simulink model "PID_Controller_referencedModel"  (R2021b)
settings: Solver=VariableStepAuto  StartTime=0.0  StopTime=10.0  RelTol=1e-3
model mask{Ki=Ki, Kp=Kp}
model workspace (MAT data in the model file):
  Kd = 1
  Ki = 1
  Kp = 1000
  Ts = 0.01
settings Model: ParameterArgumentNames=Ki,Kp  Creator=vigne  LastModifiedBy=vigne
settings DataIOCC: SaveOutput=off  SaveTime=off

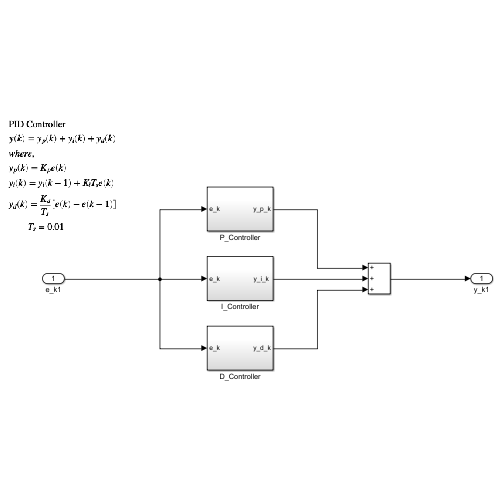
[thumbnail: Simulink's stored preview of the top-level diagram]
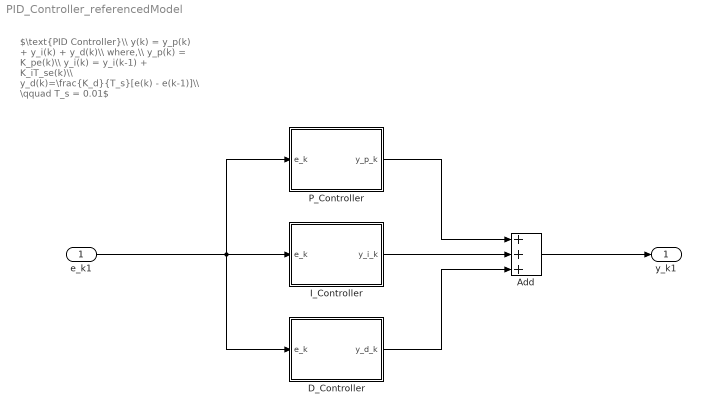
== system PID_Controller_referencedModel ==
  note: $\text{PID Controller}\\ y(k) = y_p(k) + y_i(k) + y_d(k)\\ where,\\ y_p(k) = K_pe(k)\\ y_i(k) = y_i(k-1) + K_iT_se(k)\\ y_d(k)=\frac{K_d}{T_s}[e(k) - e(k-1)]\\ \qquad T_s = 0.01$
  e_k1 : Inport  OutDataTypeStr=double  PortDimensions=1  SampleTime=0
  Add : Sum  Inputs=+++
  D_Controller : Subsystem
  I_Controller : Subsystem
  P_Controller : Subsystem
  y_k1 : Outport  OutDataTypeStr=double  PortDimensions=1  SampleTime=0
  wires:
  D_Controller/1(y_d_k) -> Add/3
  P_Controller/1(y_p_k) -> Add/1
  e_k1/1 -> P_Controller/1(e_k), D_Controller/1(e_k), I_Controller/1(e_k)
  I_Controller/1("y_i_k ") -> Add/2
  Add/1 -> y_k1/1

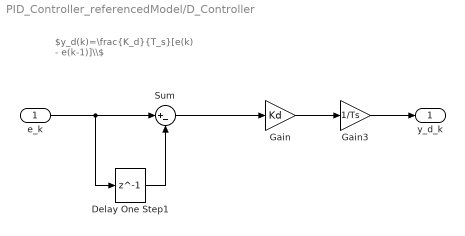
== system PID_Controller_referencedModel/D_Controller ==
  note: $y_d(k)=\frac{K_d}{T_s}[e(k) - e(k-1)]\\$
  e_k : Inport
  Delay One Step1 : Delay  DelayLength=1
  Gain : Gain  Gain=Kd
  Gain3 : Gain  Gain=1/Ts
  Sum : Sum  Inputs=|+-
  y_d_k : Outport
  wires:
  Sum/1 -> Gain/1
  Delay One Step1/1 -> Sum/2
  Gain3/1 -> y_d_k/1
  e_k/1 -> Sum/1, Delay One Step1/1
  Gain/1 -> Gain3/1

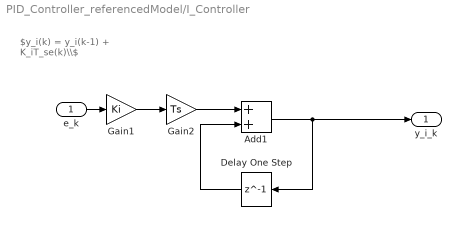
== system PID_Controller_referencedModel/I_Controller ==
  note: $y_i(k) = y_i(k-1) + K_iT_se(k)\\$
  e_k : Inport
  Add1 : Sum
  Delay One Step : Delay  DelayLength=1
  Gain1 : Gain  Gain=Ki
  Gain2 : Gain  Gain=Ts
  "y_i_k " : Outport
  wires:
  e_k/1 -> Gain1/1
  Gain2/1 -> Add1/1
  Add1/1 -> "y_i_k "/1, Delay One Step/1
  Gain1/1 -> Gain2/1
  Delay One Step/1 -> Add1/2

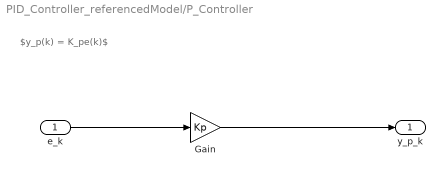
== system PID_Controller_referencedModel/P_Controller ==
  note: $y_p(k) = K_pe(k)$
  e_k : Inport
  Gain : Gain  Gain=Kp
  y_p_k : Outport
  wires:
  Gain/1 -> y_p_k/1
  e_k/1 -> Gain/1
